simulink model "untitled1"  (R2023a)
settings: Solver=FixedStepAuto  StartTime=0.0  StopTime=3  FixedStep=1e-5  RelTol=1e-3
undefined symbols (not defined in the file): J, Ki, Kiv, Kp, Kpv, KT, La, Ra, Tfi, Tfv
libraries: spsControlledVoltageSourceLib x2, spsDCMachineLib x2, spsVoltageMeasurementLib x2, sps_lib x1
settings Model: Creator=luand  LastModifiedBy=luand

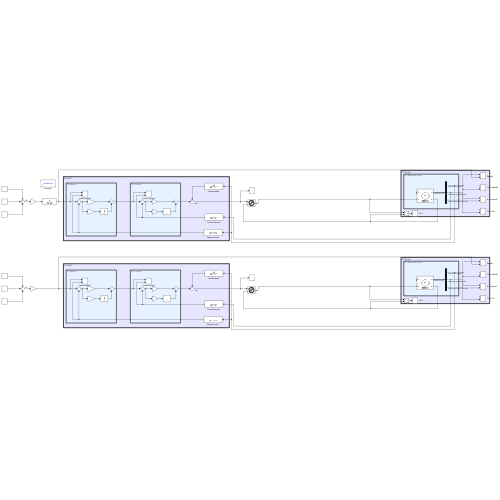
[thumbnail: Simulink's stored preview of the top-level diagram]
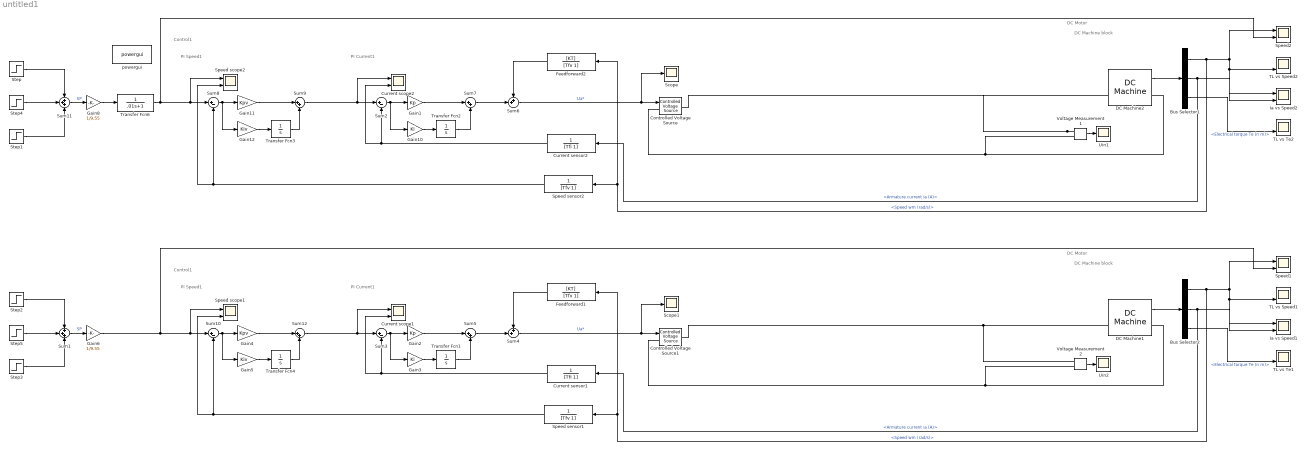
== system untitled1 ==
  note: PI Speed1
  note: PI Current1
  note: DC Motor
  note: Control1
  note: DC Machine block
  note: PI Speed1
  note: PI Current1
  note: DC Motor
  note: Control1
  note: DC Machine block
  Bus Selector1 : BusSelector  OutputSignals=Speed wm (rad/s),Armature current ia (A),Electrical torque Te (n m)
  Bus Selector2 : BusSelector  OutputSignals=Speed wm (rad/s),Armature current ia (A),Electrical torque Te (n m)
  Controlled Voltage Source : spsControlledVoltageSourceLib/Controlled Voltage Source  Initialize=on  Source_Type=DC  Amplitude=0  Phase=0  Frequency=0  Measurements=None
  Controlled Voltage Source1 : spsControlledVoltageSourceLib/Controlled Voltage Source  Initialize=on  Source_Type=DC  Amplitude=0  Phase=0  Frequency=0  Measurements=None
  Current scope1 : Scope  NumInputPorts=2
  Current scope2 : Scope  NumInputPorts=2
  Current sensor1 : TransferFcn  Denominator=[Tfi 1]
  Current sensor2 : TransferFcn  Denominator=[Tfi 1]
  DC Machine1 : spsDCMachineLib/DC Machine  PresetModel=No  MechanicalLoad=Torque TL  FieldType=Permanent magnet  ShowDetailedParameters=on  MeasurementBus=off  RLa=[ Ra La ]  RLf="[ 240  120]"  Laf=1.8  MachineConstant=Torque constant (N.m/A)  Ke=1.8  Kt=KT  J=J  Bm=0  Tf=0  w0=0  Ifinit=1  TsPowergui=0  TsBlock=-1
  DC Machine2 : spsDCMachineLib/DC Machine  PresetModel=No  MechanicalLoad=Torque TL  FieldType=Permanent magnet  ShowDetailedParameters=on  MeasurementBus=off  RLa=[ Ra La ]  RLf="[ 240  120]"  Laf=1.8  MachineConstant=Torque constant (N.m/A)  Ke=1.8  Kt=KT  J=J  Bm=0  Tf=0  w0=0  Ifinit=1  TsPowergui=0  TsBlock=-1
  Feedforward1 : TransferFcn  Numerator=[KT]  Denominator=[Tfv 1]
  Feedforward2 : TransferFcn  Numerator=[KT]  Denominator=[Tfv 1]
  Gain1 : Gain  Gain=Kp
  Gain10 : Gain  Gain=Ki
  Gain11 : Gain  Gain=Kpv
  Gain12 : Gain  Gain=Kiv
  Gain2 : Gain  Gain=Kp
  Gain3 : Gain  Gain=Ki
  Gain4 : Gain  Gain=Kpv
  Gain5 : Gain  Gain=Kiv
  Gain6 : Gain  Gain=1/9.55
  Gain8 : Gain  Gain=1/9.55
  Ia vs Speed1 : Scope  NumInputPorts=2
  Ia vs Speed2 : Scope  NumInputPorts=2
  Scope : Scope
  Scope1 : Scope
  Speed scope1 : Scope  NumInputPorts=2
  Speed scope2 : Scope  NumInputPorts=2
  Speed sensor1 : TransferFcn  Denominator=[Tfv 1]
  Speed sensor2 : TransferFcn  Denominator=[Tfv 1]
  Speed1 : Scope  NumInputPorts=2
  Speed2 : Scope  NumInputPorts=2
  Step : Step  Time=0  After=3000  SampleTime=0
  Step1 : Step  Time=2  After=-1500  SampleTime=0
  Step2 : Step  Time=0  After=3000  SampleTime=0
  Step3 : Step  Time=2  After=-1500  SampleTime=0
  Step4 : Step  After=-1500  SampleTime=0
  Step5 : Step  After=-1500  SampleTime=0
  Sum1 : Sum  Inputs=+++
  Sum{2..3,8,10} (4 alike) : Sum  Inputs=|+-
  Sum11 : Sum  Inputs=+++
  Sum{5,7,9,12} (4 alike) : Sum  Inputs=|++
  Sum4 : Sum  Inputs=++|
  Sum6 : Sum  Inputs=++|
  TL vs Speed1 : Scope  NumInputPorts=2
  TL vs Speed2 : Scope  NumInputPorts=2
  TL vs Te1 : Scope  NumInputPorts=2
  TL vs Te2 : Scope  NumInputPorts=2
  Transfer Fcn{1..4} (4 alike) : TransferFcn  Denominator=[1 0]
  Transfer Fcn6 : TransferFcn  Denominator=[.01 1]
  Uin1 : Scope
  Uin2 : Scope
  Voltage Measurement1 : spsVoltageMeasurementLib/Voltage Measurement  PhasorSimulation=off  OutputType=Complex  PSBequivalent=0
  Voltage Measurement2 : spsVoltageMeasurementLib/Voltage Measurement  PhasorSimulation=off  OutputType=Complex  PSBequivalent=0
  powergui : sps_lib/powergui  Priority=1  SimulationMode=Continuous  SampleTime=1e-5  frequency=60  Iterations=50  frequencyindice=0  Pbase=100e6  ErrMax=1e-4  UnitsV=kV  UnitsW=MW  buscounter=0  FunctionMessages=off  echomessages=off  EnableUseOfTLC=off  CurrentSourceSwitches=off  DisableSnubberDevices=off  DisableRonSwitches=off  DisableVfSwitches=off  DisplayEquations=off  AutomaticDiscreteSolvers=off  SolverType=Tustin/Backward Euler (TBE)  Interpol=off  ExternalGateDelay=off  methode=off  Ts=100  x0status=blocks  SPID=on  SwTol=0  HookPort=off  NonlinearTolerance=1e-4  nMaxIteration=100  ContinueOnMaxIteration=off  RestoreLinks=warning  ResistiveCurrentMeasurement=off  Frange=[0:2:500]  Ylog=off  Xlog=on  ShowGrid=off  save=off  variable=ZData  structure=0  ZoomFFT=off  StartTime=0.0  cycles=1  DisplayStyle=1  fundamental=60  FreqAxis=off  MaxFrequency=1000  frequencyindicesteady=1  RmsSteady=1  display=off
  wires:
  Sum2/1 -> Gain1/1, Gain10/1
  Gain11/1 -> Sum9/1
  DC Machine2/1 -> Bus Selector1/1
  Bus Selector1/1 -> Speed2/1, TL vs Speed2/2, Ia vs Speed2/2, Speed sensor2/1, Feedforward2/1  "<Speed wm (rad/s)>"
  Transfer Fcn2/1 -> Sum7/2
  Bus Selector1/3 -> TL vs Te2/2  "<Electrical torque Te (n m)>"
  Gain10/1 -> Transfer Fcn2/1
  Speed sensor2/1 -> Sum8/2, Speed scope2/2
  Current sensor2/1 -> Sum2/2, Current scope2/2
  Bus Selector1/2 -> Current sensor2/1, Ia vs Speed2/1  "<Armature current ia (A)>"
  Voltage Measurement1/1 -> Uin1/1
  Sum7/1 -> Sum6/2
  Sum9/1 -> Sum2/1, Current scope2/1
  Feedforward2/1 -> Sum6/1
  Sum6/1 -> Scope/1, Controlled Voltage Source/1  "Ua*"
  Gain1/1 -> Sum7/1
  Transfer Fcn3/1 -> Sum9/2
  Sum8/1 -> Gain11/1, Gain12/1
  Gain12/1 -> Transfer Fcn3/1
  Gain8/1 -> Transfer Fcn6/1
  Step1/1 -> Sum11/3
  Step/1 -> Sum11/1
  Sum11/1 -> Gain8/1  "SP"
  Step4/1 -> Sum11/2
  Transfer Fcn6/1 -> Speed2/2, Speed scope2/1, Sum8/1
  Gain6/1 -> Sum10/1, Speed scope1/1, Speed1/2
  Step5/1 -> Sum1/2
  Sum1/1 -> Gain6/1  "SP"
  Step2/1 -> Sum1/1
  Step3/1 -> Sum1/3
  Gain5/1 -> Transfer Fcn4/1
  Sum10/1 -> Gain5/1, Gain4/1
  Transfer Fcn4/1 -> Sum12/2
  Gain2/1 -> Sum5/1
  Sum4/1 -> Controlled Voltage Source1/1, Scope1/1  "Ua*"
  Feedforward1/1 -> Sum4/1
  Sum12/1 -> Current scope1/1, Sum3/1
  Sum5/1 -> Sum4/2
  Voltage Measurement2/1 -> Uin2/1
  Bus Selector2/2 -> Ia vs Speed1/1, Current sensor1/1  "<Armature current ia (A)>"
  Current sensor1/1 -> Current scope1/2, Sum3/2
  Speed sensor1/1 -> Speed scope1/2, Sum10/2
  Gain3/1 -> Transfer Fcn1/1
  Bus Selector2/3 -> TL vs Te1/2  "<Electrical torque Te (n m)>"
  Transfer Fcn1/1 -> Sum5/2
  Bus Selector2/1 -> Feedforward1/1, Speed sensor1/1, Ia vs Speed1/2, TL vs Speed1/2, Speed1/1  "<Speed wm (rad/s)>"
  DC Machine1/1 -> Bus Selector2/1
  Gain4/1 -> Sum12/1
  Sum3/1 -> Gain3/1, Gain2/1
  connections:
  Controlled Voltage Source/LConn1 -- Voltage Measurement1/LConn2 -- DC Machine2/RConn1
  Voltage Measurement1/LConn1 -- DC Machine2/LConn1 -- Controlled Voltage Source/RConn1
  Voltage Measurement2/LConn2 -- Controlled Voltage Source1/LConn1 -- DC Machine1/RConn1
  DC Machine1/LConn1 -- Voltage Measurement2/LConn1 -- Controlled Voltage Source1/RConn1
